simulink model "Solar_Tracking_Project"  (R2026a)
settings: Solver=VariableStepAuto  StopTime=20
InitFcn:
  | Calc;
values from neighbouring files (symbols this model uses):
  J = J_r + J_p    (= 1.001)    [Calc.m]
  K_a = 0.2    [Calc.m]
  K_b = 0.009549    [Calc.m]
  K_f = 0.047746    [Calc.m]
  N = 2    [Calc.m]
  R_m = 10    [Calc.m]
settings Model: Creator=milan  LastModifiedBy=milan

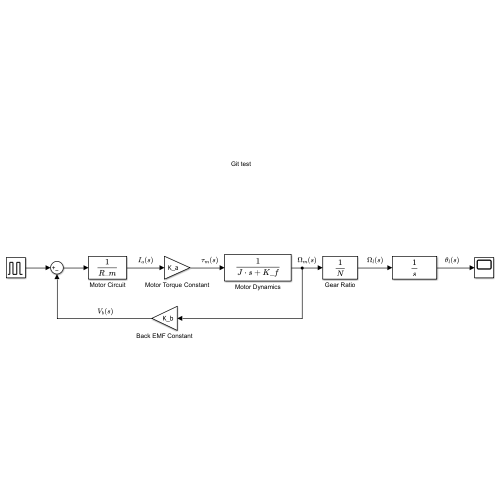
[thumbnail: Simulink's stored preview of the top-level diagram]
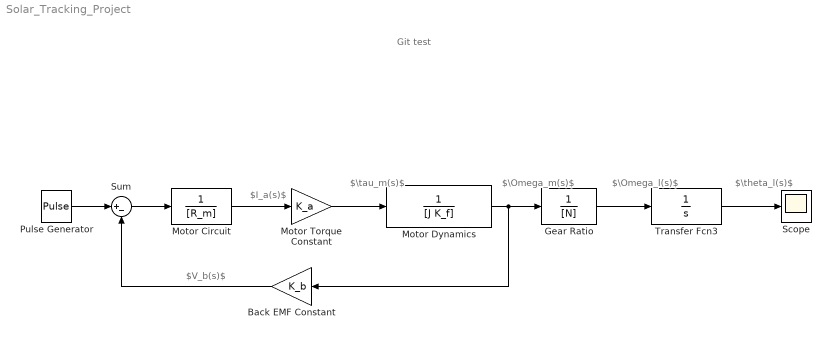
== system Solar_Tracking_Project ==
  note: Git test
  note: $V_b(s)$
  note: $I_a(s)$
  note: $\tau_m(s)$
  note: $\Omega_m(s)$
  note: $\Omega_l(s)$
  note: $\theta_l(s)$
  Back EMF Constant : Gain  Gain=K_b
  Gear Ratio : TransferFcn  Denominator=[N]
  Motor Circuit : TransferFcn  Denominator=[R_m]
  Motor Dynamics : TransferFcn  Denominator=[J K_f]
  Motor Torque Constant : Gain  Gain=K_a
  Pulse Generator : DiscretePulseGenerator  PulseType=Time based  Amplitude=20  Period=20  PulseWidth=25
  Scope : Scope
      settings: ActiveDisplayYMinimum=-3.8086259083750487  ActiveDisplayYMaximum=4.2031691228440931
  Sum : Sum  Inputs=|+-
  Transfer Fcn3 : TransferFcn  Denominator=[1 0]
  wires:
  Sum/1 -> Motor Circuit/1
  Motor Circuit/1 -> Motor Torque Constant/1
  Motor Torque Constant/1 -> Motor Dynamics/1
  Motor Dynamics/1 -> Gear Ratio/1, Back EMF Constant/1
  Back EMF Constant/1 -> Sum/2
  Gear Ratio/1 -> Transfer Fcn3/1
  Pulse Generator/1 -> Sum/1
  Transfer Fcn3/1 -> Scope/1
